simulink model "visodo10"  (Simulink 7.5)
settings: Solver=FixedStepDiscrete  StartTime=0.0  StopTime=220  FixedStep=1  RelTol=1e-3
undefined symbols (not defined in the file): gray, strel
libraries: vipsnks x2, viptextngfix x1, vipmorphops x1
(part 2 of 2)

== matlab function Matching & Visodo/Feature Uncertainty ==
  data: M input double; num_match input double; srel output double; dxyz output double
function [srel, dxyz]  = ipts_stats(M,num_match)
% function calculates statistics about ipts distribution and uncertainty


dxrel_m=zeros(1,100);
dyrel_m=zeros(1,100);
dzrel_m=zeros(1,100);
dzrel_p=zeros(1,100);
% % pred_sxrel=zeros(1,100);
srel=[0;0;0;0];
dxyz=zeros(6,100);
if num_match==0
    n=1;
else
    n=num_match;
end

% % for i=1:n
% %     xp = M(1,i); % correct for offset of camera from axle
% %     zp = M(3,i);
% %     xc = M(4,i);         
% %     zc = M(6,i);
% %     yp=M(2,i);
% %     yc=M(5,i);
% % % %     d(i)=sqrt((xc-xp)^2+(yc-yp)^2+(zc-zp)^2);
% %     dxyz(:,i)=[abs(xp-xc);xc;abs(yp-yc);yc;abs(zc-zp);zc];
% %     dxrel_m(i)=abs((xp-xc)/xc);
% %     dyrel_m(i)=abs((yp-yc)/yc);
% %     dzrel_m(i)=abs((zp-zc)/zc);
% %     dzrel_p(i)=1.4e-5*zc;
% % end
% % 
% % srel=[median(dxrel_m(1:n));median(dyrel_m(1:n));median(dzrel_m(1:n));median(dzrel_p(1:n))];

== matlab function Time/Frame Time ==
  data: el_time input double; fr_time output double
function fr_time = frame_time(el_time)
% function computes time between last frame and current frame

persistent prev_time
if isempty(prev_time)
    prev_time = 0;
end

fr_time = el_time-prev_time;

prev_time=el_time;

== matlab function Motion/Motion Plan ==
  data: L output double; R output double
function [L,R]=motion()

% function generates oval motion
persistent c_pers
if isempty(c_pers)
    c_pers=0;
end

R=1.0;
L=1.0;

c=c_pers;

% define number of steps for straightaway & turn
str=60;
turn=70;

if c<=str
    c=c+1;
    L=1.0;
    
elseif c>str && c<str+turn
    c=c+1;
    L=.4;
    R=1.6;
    
elseif c>=turn
    c=0;
    L=1.0;
end

c_pers=c;
% % L=0.4;
% % R=1.6;

== matlab function Matching & Visodo/Store Match History ==
  data: M_hist_vec output double; M_rpix_hist_vec output double; M input double; M_hist output double; num_match input double; M_rpix_hist output double; M_rpix input double
function [M_hist_vec,M_rpix_hist_vec,M_hist,M_rpix_hist]=match_hist(M, num_match, M_rpix)
% functions stores history of matches

persistent M_hist_pers index_pers next_col_pers M_rpix_hist_pers index_rpix_pers
if isempty(M_hist_pers)
    M_hist_pers = zeros(666,20);
    M_rpix_hist_pers=zeros(2*221,20);
    
    index_pers=zeros(1,20); % vector of last row entry in each column
    index_rpix_pers=zeros(1,20);
    next_col_pers=0;
end

M_hist_vec=zeros(666*20,1);
M_rpix_hist_vec=zeros(2*221*20,1);

M_hist=M_hist_pers;
M_rpix_hist=M_rpix_hist_pers;
index=index_pers;
index_rpix=index_rpix_pers;
next_col=next_col_pers;

if num_match>0

    for p=1:20 % loop through previous entries
        if index(p)==0
            M_hist(1:6,p)=M(1:6,p);
            index(p)=7;
            M_rpix_hist(1:2,p)=M_rpix(1:2,p);
            index_rpix(p)=3;
        else
            for c=1:num_match
                if sum(M(1:3,c)-M_hist(index(p)-3:index(p)-1,p))==0 %%ie, if current is in history
                    M_hist(index(p):index(p)+2,p)=M(4:6,c);
                    index(p)=index(p)+3;
                    
                    M_rpix_hist(index_rpix(p):index_rpix(p)+1,p)=M_rpix(1:2,c);
                    index_rpix(p)=index_rpix(p)+2;
                
                end
            end
        end
    end

end
% convert M_hist to vector for storing output
i=0;
j=0;
for c=1:20
    for r=1:666
        i=i+1;
        M_hist_vec(i,1)=M_hist(r,c);
    end
    for rp=1:442
        j=j+1;
        M_rpix_hist_vec(j,1)=M_rpix_hist(rp,c);
    end
end

next_col_pers=next_col;
index_pers=index;
M_hist_pers=M_hist;
index_rpix_pers=index_rpix;
M_rpix_hist_pers=M_rpix_hist;

== matlab function Motion/Motor Control/Embedded MATLAB Function1 ==
  data: M1in input double; M1 output double; M2in input double; M2 output double
function [M1, M2] = MotorPackets(M1in, M2in)
%#eml

M1 = 0;
M2 = 1;

if M1in <= 0
    M1 = M1+2;
end

if M2in <= 0
    M2 = M2+2;
end

M1 = M1 + round(abs(M1in)*10)*4;
M2 = M2 + round(abs(M2in)*10)*4;
